simulink model "Bernoulli"  (R2021a)
settings: Solver=ode45  StartTime=0.0  StopTime=10000  RelTol=1e-3  EnableMultiTasking=on
libraries: commsink2 x2, commcrc2 x2, commrandsrc2 x1, commchan3 x1, dspswit3 x1
settings Model: Creator=student  LastModifiedBy=vitak
settings SolverCC: AlgebraicLoopSolver=TrustRegion
settings DataIOCC: LimitDataPoints=on  SaveFormat=Array  ReturnWorkspaceOutputs=off
settings OptimizationCC: InitFltsAndDblsToZero=on  LifeSpan=inf
settings DebuggingCC: SaveWithParameterizedLinksMsg=none  UnderspecifiedInitializationDetection=Classic  MergeDetectMultiDrivingBlocksExec=none  SignalResolutionControl=TryResolveAllWithWarning  SolverPrmCheckMsg=warning  MultiTaskDSMMsg=warning  MultiTaskCondExecSysMsg=none  FcnCallInpInsideContextMsg=warning  AllowSymbolicDim=off  SFUnexpectedBacktrackingDiag=warning  SFNoUnconditionalDefaultTransitionDiag=warning  SFExecutionAtInitializationDiag=none  SFMachineParentedDataDiag=warning  ArithmeticOperatorsInVariantConditions=warning
settings HardwareCC: ProdBitPerPointer=32  ProdBitPerSizeT=32  ProdBitPerPtrDiffT=32  ProdLargestAtomicFloat=None  ProdIntDivRoundTo=Undefined  ProdEndianess=Unspecified  ProdWordSize=32  ProdHWDeviceType=32-bit Generic
settings ModelReferenceCC: PropagateSignalLabelsOutOfModel=off
settings SFSimCC: SimUseLocalCustomCode=off  CustomCodeUndefinedFunction=UseInterfaceOnly
settings RTWCC: RTWUseLocalCustomCode=off
settings CodeAppCC: StateflowObjectComments=on
settings GRTTargetCC: TargetFcnLib=ansi_tfl_tmw.mat  TargetLangStandard=C89/C90 (ANSI)  CombineOutputUpdateFcns=off  GRTInterface=on
settings ConfigComp: CovMetricSettings=dw  CovSaveCumulativeToWorkspaceVar=on  CovSaveSingleToWorkspaceVar=on  CovExternalEMLEnable=off

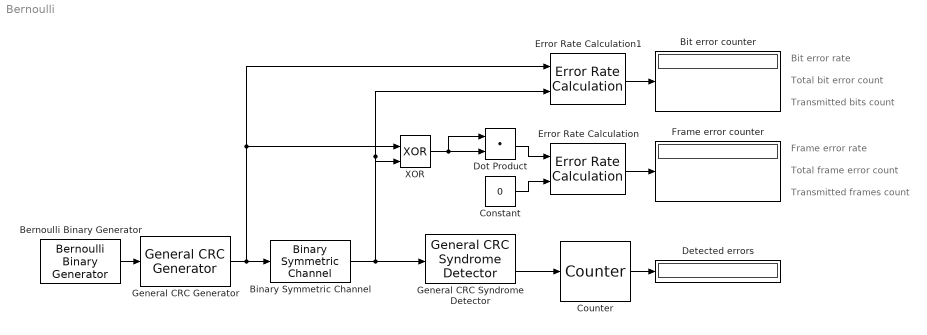
== system Bernoulli ==
  note: Frame error rate
  note: Total frame error count
  note: Transmitted frames count
  note: Transmitted bits count
  note: Bit error rate
  note: Total bit error count
  Bernoulli Binary Generator : commrandsrc2/Bernoulli Binary Generator  P=0.5  seed=0  Ts=1/3000  frameBased=on  sampPerFrame=100  orient=off  outDataType=double
      settings: SourceProductBaseCode=CM
  Binary Symmetric Channel : commchan3/Binary Symmetric Channel  ErrorProbability=0.01  ErrorVectorOutputPort=off  OutputDataType=double  OutputDataTypeSL=double  Seed=0  SimulateUsing=Code generation
      settings: SourceProductBaseCode=CM
  Bit error counter : Display
  Constant : Constant  Value=0  OutDataTypeStr=uint16
  Counter : dspswit3/Counter  Direction=Up  CountEvent=Non-zero sample  CounterSize=User defined  MaxCount=65535000  InitialCount=0  Output=Count  HitValue=32  ResetInput=off  SamplesPerFrame=1  Ts=1  CntDtype=double  HitDtype=Logical
  Detected errors : Display
  Dot Product : DotProduct  InputSameDT=on  OutDataTypeStr=Inherit: Inherit via internal rule
  Error Rate Calculation : commsink2/Error Rate Calculation  N=0  st_delay=0  cp_mode=Entire frame  subframe=[]  PMode=Port  WsName=ErrorVec  RsMode2=off  stop=off  numErr=100  maxBits=1e6
  Error Rate Calculation1 : commsink2/Error Rate Calculation  N=0  st_delay=0  cp_mode=Entire frame  subframe=[]  PMode=Port  WsName=ErrorVec  RsMode2=off  stop=off  numErr=100  maxBits=1e6
  Frame error counter : Display
  General CRC Generator : commcrc2/General CRC Generator  genPoly=[1 1 1 0 1 0 1 0 1]  iniStates=[0]  directMethod=off  reflectInputBytes=off  reflectChecksums=off  finalXOR=0  numChecksums=1
      settings: SourceProductBaseCode=CM
  General CRC Syndrome Detector : commcrc2/General CRC Syndrome Detector  genPoly=[1 1 1 0 1 0 1 0 1]  iniStates=[0]  directMethod=off  reflectInputBytes=off  reflectChecksums=off  finalXOR=0  numChecksums=1
      settings: SourceProductBaseCode=CM
  XOR : Logic  Operator=XOR  IconShape=distinctive  AllPortsSameDT=off  OutDataTypeStr=boolean
  wires:
  Counter/1 -> Detected errors/1
  Bernoulli Binary Generator/1 -> General CRC Generator/1
  General CRC Generator/1 -> Error Rate Calculation1/1, XOR/1, Binary Symmetric Channel/1
  Binary Symmetric Channel/1 -> Error Rate Calculation1/2, XOR/2, General CRC Syndrome Detector/1
  General CRC Syndrome Detector/2 -> Counter/1
  Error Rate Calculation/1 -> Frame error counter/1
  Dot Product/1 -> Error Rate Calculation/1
  Constant/1 -> Error Rate Calculation/2
  XOR/1 -> Dot Product/1, Dot Product/2
  Error Rate Calculation1/1 -> Bit error counter/1
